simulink model "prob9_"  (R2020b)
settings: Solver=VariableStepAuto  StartTime=0.0  StopTime=10.0  RelTol=1e-3
values from neighbouring files (symbols this model uses):
  kf = 4    [matlab.mat]
  Te = 5    [matlab.mat]
  TL = 4    [matlab.mat]
undefined symbols (not defined in the file or in its folder): J
settings Model: Creator=Pulkit Khandelwal  LastModifiedBy=Pulkit Khandelwal

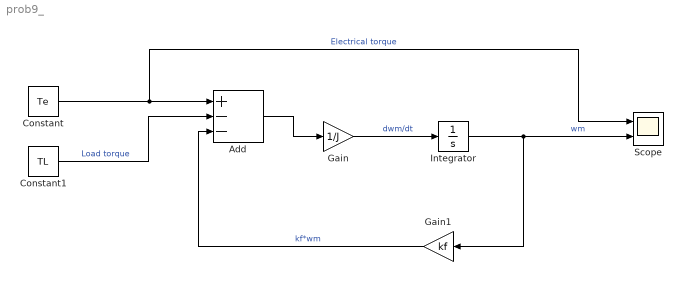
== system prob9_ ==
  Add : Sum  Inputs=+--
  Constant : Constant  Value=Te
  Constant1 : Constant  Value=TL
  Gain : Gain  Gain=1/J
  Gain1 : Gain  Gain=kf
  Integrator : Integrator
  Scope : Scope  NumInputPorts=2
  wires:
  Gain/1 -> Integrator/1  "dwm/dt"
  Add/1 -> Gain/1
  Integrator/1 -> Gain1/1, Scope/2  "wm"
  Gain1/1 -> Add/3  "kf*wm"
  Constant/1 -> Scope/1, Add/1  "Electrical torque"
  Constant1/1 -> Add/2  "Load torque"
